simulink model "torqueBalancingPHRIStandup_WBTv5"  (Simulink 9.1)
settings: Solver=FixedStepDiscrete  StartTime=0.0  StopTime="Config.SIMULATION_TIME "  FixedStep=Config.Ts  RelTol=1e-3  EnableMultiTasking=on
StopFcn:
  | cd(fileparts(which(bdroot)));
  | stopTorqueBalancingPHRIStandup;
undefined symbols (not defined in the file or in its folder): ASSISTANT_DOF_FOR_SIMULINK, bVectorConstraintsFeet, bVectorConstraintsLegs, Config, ConstraintsMatrixFeet, ConstraintsMatrixLegs, DiscIntNeverNeededParam, Gain, Reg, ROBOT_DOF, ROBOT_DOF_FOR_SIMULINK, Sat, Sm
libraries: WBToolboxLibrary x155, simulink x5
(part 3 of 4)

== system torqueBalancingPHRIStandup_WBTv5/Robot system/Robot State and References/Internal Coordinator/Base to fixed_link ==
  qj : Inport
  inertial : Inport  Port=2
  Constant1 : Constant  Value=Config.LEFT_FOOT_IN_CONTACT_AT_0
  Constant7 : Constant  Value=eye(4)
  "LFoot to base link transform " : Subsystem
  LFoot to world transform (fixed base) : WBToolboxLibrary/Model/Kinematics/ForwardKinematics  frameName=Frames.LEFT_FOOT
      settings: SourceProductName=WholeBodyToolbox
  RFoot to world transform (fixed base) : WBToolboxLibrary/Model/Kinematics/ForwardKinematics  frameName=Frames.RIGHT_FOOT
      settings: SourceProductName=WholeBodyToolbox
  Switch : Switch  Criteria=u2 > Threshold
  fixed_LFoot_H_b : Outport
  wires:
  "LFoot to base link transform "/1(link_H_b) -> fixed_LFoot_H_b/1
  inertial/1 -> "LFoot to base link transform "/2(inertial)
  qj/1 -> "LFoot to base link transform "/1(qj), RFoot to world transform (fixed base)/2, LFoot to world transform (fixed base)/2
  Constant7/1 -> LFoot to world transform (fixed base)/1, RFoot to world transform (fixed base)/1, "LFoot to base link transform "/4(w_H_base_fixed)
  Switch/1 -> "LFoot to base link transform "/3(w_H_link)
  LFoot to world transform (fixed base)/1 -> Switch/1
  RFoot to world transform (fixed base)/1 -> Switch/3
  Constant1/1 -> Switch/2

== system torqueBalancingPHRIStandup_WBTv5/Robot system/Robot State and References/Internal Coordinator/Compute State Velocity ==
  qj : Inport
  w_H_b : Inport  Port=2
  "feetInContact " : Inport  Port=3
  Compute Base Velocity : MATLAB Function  TreatAsAtomicUnit=on
  Feet Jacobians : Subsystem
  GetMeasurement : WBToolboxLibrary/States/GetMeasurement  measuredType=Joints Velocity
      settings: SourceProductName=WholeBodyToolbox
  Mux : Mux  Inputs=2
  nu : Outport
  wires:
  GetMeasurement/1 -> Mux/2, Compute Base Velocity/4(qjDot)
  Mux/1 -> nu/1
  "feetInContact "/1 -> Compute Base Velocity/3(feetInContact)
  Compute Base Velocity/1(nu_b) -> Mux/1
  qj/1 -> Feet Jacobians/1(qj)
  w_H_b/1 -> Feet Jacobians/2(w_H_b)
  Feet Jacobians/1(J_LFoot) -> Compute Base Velocity/1(J_LeftFoot)
  Feet Jacobians/2(J_RFoot) -> Compute Base Velocity/2(J_RightFoot)

== system torqueBalancingPHRIStandup_WBTv5/Robot system/Robot State and References/Internal Coordinator/xCom ==
  w_H_b : Inport
  qj : Inport  Port=2
  CoM : WBToolboxLibrary/Model/Kinematics/ForwardKinematics  frameName=Frames.COM
      settings: SourceProductName=WholeBodyToolbox
  "CoM6D ->  CoMXYZ2" : Selector  NumberOfDimensions=2  InputPortWidth=7  IndexOptions=Index vector (dialog),Index vector (dialog)  Indices=[1 2 3],[4]  OutputSizes=1,1
  xCoM : Outport
  wires:
  qj/1 -> CoM/2
  "CoM6D ->  CoMXYZ2"/1 -> xCoM/1
  CoM/1 -> "CoM6D ->  CoMXYZ2"/1
  w_H_b/1 -> CoM/1

== system torqueBalancingPHRIStandup_WBTv5/Robot system/Robot State and References/Select State and References/Simulink Min-jerk Trajectory  ==
  CoMDes : Inport
  smoothingTimeMinJerkComDesQDes : Inport  Port=2
  MinimumJerkTrajectoryGenerator2 : WBToolboxLibrary/Utilities/MinimumJerkTrajectoryGenerator  externalSettlingTime=on  settlingTime=0.1  sampleTime=Config.Ts  resetOnSettlingTime=off  firstDerivatives=on  secondDerivatives=on  explicitInitialValue=off
      settings: SourceProductName=WholeBodyToolbox
  Mux : Mux  Inputs=3
  Selector : Selector  InputPortWidth=9  IndexOptions=Index vector (dialog)  Indices=[1 2 3]  OutputSizes=1
  Switch1 : Switch  Criteria=u2 > Threshold
  Switch3 : Switch  Criteria=u2 > Threshold
  joints.smoothingTime : Constant  Value=Sm.smoothingTimeCoM
  desired_x_dx_ddx_CoM : Outport
  wires:
  Switch1/1 -> MinimumJerkTrajectoryGenerator2/2
  MinimumJerkTrajectoryGenerator2/2 -> Mux/2
  joints.smoothingTime/1 -> Switch1/3
  Mux/1 -> Switch3/1
  Switch3/1 -> desired_x_dx_ddx_CoM/1
  smoothingTimeMinJerkComDesQDes/1 -> Switch1/1, Switch1/2, Switch3/2
  MinimumJerkTrajectoryGenerator2/3 -> Mux/3
  Selector/1 -> MinimumJerkTrajectoryGenerator2/1
  MinimumJerkTrajectoryGenerator2/1 -> Mux/1
  CoMDes/1 -> Switch3/3, Selector/1

== system torqueBalancingPHRIStandup_WBTv5/Robot system/Robot State and References/Select State and References/Visualize Gain Tuning   ==
  smoothingTimeComAndJoints : Inport
  LEFT_RIGHT_FOOT_IN_CONTACT : Inport  Port=2
  impedances : Inport  Port=3
  state : Inport  Port=4
  nu : Inport  Port=5
  Enable : EnablePort
  Demux : Demux  Outputs=2
  DoFs converter : WBToolboxLibrary/Utilities/DoFs converter  Commented=on  yarp2WBIOption=From YARP to WBI
      settings: SourceProductName=WholeBodyToolbox
  DoFs converter1 : WBToolboxLibrary/Utilities/DoFs converter  Commented=on  yarp2WBIOption=From YARP to WBI
      settings: SourceProductName=WholeBodyToolbox
  Gain : Gain  Gain=180/pi
  Gain1 : Gain  Gain=180/pi
  Impedances(t) : Scope  Commented=on  NumInputPorts=6
  Left right foot in contact : Scope
  Selector1 : Selector  InputPortWidth=6+ROBOT_DOF  IndexOptions=Index vector (dialog)  Indices=[7:6+ROBOT_DOF]  OutputSizes=1
  Selector2 : Selector  InputPortWidth=6+ROBOT_DOF  IndexOptions=Index vector (dialog)  Indices=[1:6]  OutputSizes=1
  jointsSmoothingTime : Scope  NumInputPorts=2
  linear and angular  base velocity : Scope  NumInputPorts=3
  "qjDot(t) " : Scope  Commented=on  NumInputPorts=6
  wires:
  state/1 -> "qjDot(t) "/6, linear and angular  base velocity/3, Impedances(t)/6, jointsSmoothingTime/2  "state"
  LEFT_RIGHT_FOOT_IN_CONTACT/1 -> Left right foot in contact/1  "Left right foot in contact"
  impedances/1 -> DoFs converter/1
  smoothingTimeComAndJoints/1 -> jointsSmoothingTime/1  "smoothingTimeComAndJoints"
  DoFs converter/4 -> Impedances(t)/4  "left_leg"
  DoFs converter/5 -> Impedances(t)/5  "right_leg"
  DoFs converter/3 -> Impedances(t)/3  "right_arm"
  DoFs converter/1 -> Impedances(t)/1  "torso"
  DoFs converter/2 -> Impedances(t)/2  "left_arm"
  Selector1/1 -> Gain/1
  DoFs converter1/4 -> "qjDot(t) "/4  "left_leg"
  DoFs converter1/3 -> "qjDot(t) "/3  "right_arm"
  DoFs converter1/1 -> "qjDot(t) "/1  "torso"
  DoFs converter1/2 -> "qjDot(t) "/2  "left_arm"
  nu/1 -> Selector2/1, Selector1/1
  Selector2/1 -> Demux/1
  Demux/1 -> linear and angular  base velocity/1  "vb"
  Demux/2 -> Gain1/1  "wb"
  Gain/1 -> DoFs converter1/1
  Gain1/1 -> linear and angular  base velocity/2
  DoFs converter1/5 -> "qjDot(t) "/5  "right_leg"

== system torqueBalancingPHRIStandup_WBTv5/Robot system/Robot State and References/State Machine Standup/Compute State Velocity ==
  qj : Inport
  w_H_b : Inport  Port=2
  "feetInContact " : Inport  Port=3
  "state " : Inport  Port=4
  Compute Base Velocity : MATLAB Function  TreatAsAtomicUnit=on
  Fixed Links Jacobians : Subsystem
  GetMeasurement : WBToolboxLibrary/States/GetMeasurement  measuredType=Joints Velocity
      settings: SourceProductName=WholeBodyToolbox
  Mux : Mux  Inputs=2
  nu : Outport
  wires:
  GetMeasurement/1 -> Mux/2, Compute Base Velocity/4(qjDot)
  Mux/1 -> nu/1
  "feetInContact "/1 -> Compute Base Velocity/3(feetInContact)
  Compute Base Velocity/1(nu_b) -> Mux/1
  Fixed Links Jacobians/1(J_LeftFixed) -> Compute Base Velocity/1(J_LeftFixedLink)
  Fixed Links Jacobians/2(J_RightFixed) -> Compute Base Velocity/2(J_RightFixedLink)
  "state "/1 -> Fixed Links Jacobians/1("state ")
  qj/1 -> Fixed Links Jacobians/2(qj)
  w_H_b/1 -> Fixed Links Jacobians/3(w_H_b)

== system torqueBalancingPHRIStandup_WBTv5/Robot system/Robot State and References/State Machine Standup/Compute base to fixed link transform ==
  qj : Inport
  inertial : Inport  Port=2
  Constant7 : Constant  Value=eye(4)
  "LFoot to base link transform " : Subsystem
  LFoot to world transform (fixed base) : WBToolboxLibrary/Model/Kinematics/ForwardKinematics  frameName=Frames.LEFT_FOOT
      settings: SourceProductName=WholeBodyToolbox
  LLeg to base link transform : Subsystem
  LLeg to world transform (fixed base) : WBToolboxLibrary/Model/Kinematics/ForwardKinematics  frameName=Frames.LEFT_LEG
      settings: SourceProductName=WholeBodyToolbox
  fixed_LFoot_H_b : Outport
  fixed_LLeg_H_b : Outport  Port=2
  wires:
  Constant7/1 -> LLeg to base link transform/4(w_H_base_fixed), "LFoot to base link transform "/4(w_H_base_fixed), LLeg to world transform (fixed base)/1, LFoot to world transform (fixed base)/1
  LLeg to base link transform/1(link_H_b) -> fixed_LLeg_H_b/1
  "LFoot to base link transform "/1(link_H_b) -> fixed_LFoot_H_b/1
  LFoot to world transform (fixed base)/1 -> "LFoot to base link transform "/3(w_H_link)
  LLeg to world transform (fixed base)/1 -> LLeg to base link transform/3(w_H_link)
  qj/1 -> "LFoot to base link transform "/1(qj), LLeg to base link transform/1(qj), LLeg to world transform (fixed base)/2, LFoot to world transform (fixed base)/2
  inertial/1 -> "LFoot to base link transform "/2(inertial), LLeg to base link transform/2(inertial)

== system torqueBalancingPHRIStandup_WBTv5/Robot system/Robot State and References/State Machine Standup/Visualise extrnal wrenches ==
  wL_arm : Inport
  wR_arm : Inport  Port=2
  wL_WBDT : Inport  Port=3
  wR_WBDT : Inport  Port=4
  state : Inport  Port=5
  Enable : EnablePort
  Compute current threshold : MATLAB Function  TreatAsAtomicUnit=on
  Sum : Sum  Inputs=++|
  Sum1 : Sum  Inputs=++|
  left arm ext wrench : Scope  NumInputPorts=3
  left foot ext wrench : Scope  NumInputPorts=3
  right arm ext wrench : Scope  NumInputPorts=3
  right foot ext wrench : Scope  NumInputPorts=3
  sum feet ext wrench : Scope  NumInputPorts=3
  wires:
  wR_WBDT/1 -> Sum/2, right foot ext wrench/1  "wR_WBDT"
  wL_WBDT/1 -> Sum/1, left foot ext wrench/1  "wL_WBDT"
  wR_arm/1 -> right arm ext wrench/1
  wL_arm/1 -> left arm ext wrench/1
  state/1 -> Compute current threshold/1(state), sum feet ext wrench/3, right foot ext wrench/3, left foot ext wrench/3, right arm ext wrench/3, left arm ext wrench/3
  Sum/1 -> sum feet ext wrench/1
  Sum1/1 -> sum feet ext wrench/2
  Compute current threshold/3(thresholdContactLeftFoot) -> left foot ext wrench/2, Sum1/1
  Compute current threshold/4(thresholdContactRightFoot) -> right foot ext wrench/2, Sum1/2
  Compute current threshold/1(thresholdContactLeftHand) -> left arm ext wrench/2
  Compute current threshold/2(thresholdContactRightHand) -> right arm ext wrench/2

== system torqueBalancingPHRIStandup_WBTv5/Robot system/Robot State and References/State Machine Standup/xCom ==
  w_H_b : Inport
  qj : Inport  Port=2
  CoM : WBToolboxLibrary/Model/Kinematics/ForwardKinematics  frameName=Frames.COM
      settings: SourceProductName=WholeBodyToolbox
  "CoM6D ->  CoMXYZ2" : Selector  NumberOfDimensions=2  InputPortWidth=7  IndexOptions=Index vector (dialog),Index vector (dialog)  Indices=[1 2 3],[4]  OutputSizes=1,1
  xCoM : Outport
  wires:
  qj/1 -> CoM/2
  "CoM6D ->  CoMXYZ2"/1 -> xCoM/1
  CoM/1 -> "CoM6D ->  CoMXYZ2"/1
  w_H_b/1 -> CoM/1

== system torqueBalancingPHRIStandup_WBTv5/Robot system/controller_QP/Compute angular momentum integral/Compute base to fixed link transform ==
  qj : Inport
  inertial : Inport  Port=2
  Constant7 : Constant  Value=eye(4)
  "LFoot to base link transform " : Subsystem
  LFoot to world transform (fixed base) : WBToolboxLibrary/Model/Kinematics/ForwardKinematics  frameName=Frames.LEFT_FOOT
      settings: SourceProductName=WholeBodyToolbox
  LLeg to base link transform : Subsystem
  LLeg to world transform (fixed base) : WBToolboxLibrary/Model/Kinematics/ForwardKinematics  frameName=Frames.LEFT_LEG
      settings: SourceProductName=WholeBodyToolbox
  fixed_LLeg_H_b : Outport
  fixed_LFoot_H_b : Outport  Port=2
  wires:
  Constant7/1 -> LLeg to base link transform/4(w_H_base_fixed), "LFoot to base link transform "/4(w_H_base_fixed), LLeg to world transform (fixed base)/1, LFoot to world transform (fixed base)/1
  LLeg to base link transform/1(link_H_b) -> fixed_LLeg_H_b/1
  "LFoot to base link transform "/1(link_H_b) -> fixed_LFoot_H_b/1
  LFoot to world transform (fixed base)/1 -> "LFoot to base link transform "/3(w_H_link)
  LLeg to world transform (fixed base)/1 -> LLeg to base link transform/3(w_H_link)
  qj/1 -> "LFoot to base link transform "/1(qj), LLeg to base link transform/1(qj), LLeg to world transform (fixed base)/2, LFoot to world transform (fixed base)/2
  inertial/1 -> "LFoot to base link transform "/2(inertial), LLeg to base link transform/2(inertial)

== system torqueBalancingPHRIStandup_WBTv5/Robot system/controller_QP/Compute angular momentum integral/Fixed Links Jacobians ==
  "legsInContact " : Inport
  qj : Inport  Port=2
  w_H_b : Inport  Port=3
  " " : WBToolboxLibrary/Model/Jacobians/Jacobian  frameName=Frames.LEFT_LEG
      settings: SourceProductName=WholeBodyToolbox
  "  " : WBToolboxLibrary/Model/Jacobians/Jacobian  frameName=Frames.RIGHT_LEG
      settings: SourceProductName=WholeBodyToolbox
  "   " : WBToolboxLibrary/Model/Jacobians/Jacobian  frameName=Frames.RIGHT_FOOT
      settings: SourceProductName=WholeBodyToolbox
  "       " : WBToolboxLibrary/Model/Jacobians/Jacobian  frameName=Frames.LEFT_FOOT
      settings: SourceProductName=WholeBodyToolbox
  Switch1 : Switch  Criteria=u2 > Threshold  Threshold=0.1
  Switch2 : Switch  Criteria=u2 > Threshold  Threshold=0.1
  J_LeftFixed : Outport
  J_RIghtFixed : Outport  Port=2
  wires:
  Switch2/1 -> J_RIghtFixed/1
  " "/1 -> Switch1/1
  "       "/1 -> Switch1/3
  "   "/1 -> Switch2/3
  "  "/1 -> Switch2/1
  Switch1/1 -> J_LeftFixed/1
  qj/1 -> "   "/2, "  "/2, "       "/2, " "/2
  w_H_b/1 -> "   "/1, " "/1, "       "/1, "  "/1
  "legsInContact "/1 -> Switch2/2, Switch1/2

== system torqueBalancingPHRIStandup_WBTv5/Robot system/controller_QP/Compute joint torques/QPSolver ==
  LEFT_RIGHT_FOOT_IN_CONTACT : Inport
  HessianMatrixQP1Foot : Inport  Port=2
  gradientQP1Foot : Inport  Port=3
  ConstraintsMatrixQP1Foot : Inport  Port=4
  bVectorConstraintsQP1Foot : Inport  Port=5
  HessianMatrixQP2Feet : Inport  Port=6
  gradientQP2Feet : Inport  Port=7
  ConstraintsMatrixQP2Feet : Inport  Port=8
  bVectorConstraintsQp2Feet : Inport  Port=9
  state : Inport  Port=10
  Constant1 : Constant  Value=Config.USE_QP_SOLVER
  Level-2 MATLAB S-Function : M-S-Function  FunctionName=QPBalancingStandup
  Logical Operator1 : Logic  Operator=OR  AllPortsSameDT=off  OutDataTypeStr=boolean
  ON_GAZEBO 3 : Constant  Value=Config.SCOPES_ALL
  ON_GAZEBO 4 : Constant  Value=Config.SCOPES_QP
  Visualize eventual QP failures : Subsystem
  f0OneFoot : Outport
  f0TwoFeet : Outport  Port=2
  wires:
  Level-2 MATLAB S-Function/1 -> f0TwoFeet/1
  Level-2 MATLAB S-Function/2 -> Visualize eventual QP failures/1(exitFlagQP)  "Exit flag QP two feet"
  HessianMatrixQP1Foot/1 -> Level-2 MATLAB S-Function/7
  gradientQP1Foot/1 -> Level-2 MATLAB S-Function/8
  ConstraintsMatrixQP1Foot/1 -> Level-2 MATLAB S-Function/9
  bVectorConstraintsQP1Foot/1 -> Level-2 MATLAB S-Function/10
  Level-2 MATLAB S-Function/3 -> f0OneFoot/1
  Logical Operator1/1 -> Visualize eventual QP failures/Enable
  state/1 -> Visualize eventual QP failures/2(state)
  LEFT_RIGHT_FOOT_IN_CONTACT/1 -> Level-2 MATLAB S-Function/1
  HessianMatrixQP2Feet/1 -> Level-2 MATLAB S-Function/2
  gradientQP2Feet/1 -> Level-2 MATLAB S-Function/3
  ConstraintsMatrixQP2Feet/1 -> Level-2 MATLAB S-Function/4
  bVectorConstraintsQp2Feet/1 -> Level-2 MATLAB S-Function/5
  Constant1/1 -> Level-2 MATLAB S-Function/6
  ON_GAZEBO 3/1 -> Logical Operator1/1
  ON_GAZEBO 4/1 -> Logical Operator1/2

== system torqueBalancingPHRIStandup_WBTv5/Assistant system/Real system/Dump and visualize/Assistant Data/Using Human Assistant ==
  assistant_jointData : Inport
  assistant_jointVelocitiesData : Inport  Port=2
  assistant_jointTorquesData : Inport  Port=3
  Enable : EnablePort
  Gain : Gain  Gain=180/pi
  Gain1 : Gain  Gain=180/pi
  assistant joint data : Subsystem
  assistant joint torques data : Subsystem
  assistant joint velocities data : Subsystem
  wires:
  Gain/1 -> assistant joint data/1(assistant_jointData)
  assistant_jointData/1 -> Gain/1
  Gain1/1 -> assistant joint velocities data/1(assistant_jointVelocitiesData)
  assistant_jointVelocitiesData/1 -> Gain1/1
  assistant_jointTorquesData/1 -> assistant joint torques data/1(assistant_jointTorquesData)

== system torqueBalancingPHRIStandup_WBTv5/Assistant system/Real system/Dump and visualize/Assistant Data/Using Robot Assistant ==
  assistant_jointData : Inport
  assistant_jointVelocitiesData : Inport  Port=2
  assistant_jointTorquesData : Inport  Port=3
  Enable : EnablePort
  Demux1 : Demux  Outputs=ASSISTANT_Config.numOfJointsForEachControlboard
  Demux2 : Demux  Outputs=ASSISTANT_Config.numOfJointsForEachControlboard
  Demux3 : Demux  Outputs=ASSISTANT_Config.numOfJointsForEachControlboard
  scope : Scope  NumInputPorts=5
  scope1 : Scope  NumInputPorts=5
  scope2 : Scope  NumInputPorts=5
  wires:
  Demux1/1 -> scope/1  "torso"
  Demux1/5 -> scope/5  "rightleg"
  Demux1/4 -> scope/4  "left_leg"
  assistant_jointData/1 -> Demux1/1
  Demux1/2 -> scope/2  "left_arm"
  Demux1/3 -> scope/3  "right_arm"
  Demux2/5 -> scope1/5  "rightleg"
  assistant_jointVelocitiesData/1 -> Demux2/1
  Demux2/4 -> scope1/4  "left_leg"
  Demux2/1 -> scope1/1  "torso"
  Demux2/2 -> scope1/2  "left_arm"
  Demux2/3 -> scope1/3  "right_arm"
  Demux3/5 -> scope2/5  "rightleg"
  assistant_jointTorquesData/1 -> Demux3/1
  Demux3/4 -> scope2/4  "left_leg"
  Demux3/1 -> scope2/1  "torso"
  Demux3/2 -> scope2/2  "left_arm"
  Demux3/3 -> scope2/3  "right_arm"

== system torqueBalancingPHRIStandup_WBTv5/Robot system/Robot State and References/Internal Coordinator/Base to fixed_link/LFoot to base link transform  ==
  qj : Inport
  inertial : Inport  Port=2
  w_H_link : Inport  Port=3
  w_H_base_fixed : Inport  Port=4
  Fixed base to imu transform : WBToolboxLibrary/Model/Kinematics/ForwardKinematics  frameName=Frames.IMU
      settings: SourceProductName=WholeBodyToolbox
  Fixed base to root link transform : WBToolboxLibrary/Model/Kinematics/ForwardKinematics  frameName=Frames.BASE
      settings: SourceProductName=WholeBodyToolbox
  Inv\* : Product  Inputs=/*  Multiplication=Matrix(*)
  "Inv\\*  " : Product  Inputs=/*  Multiplication=Matrix(*)
  Neck Position : WBToolboxLibrary/Utilities/YarpRead  portName=Ports.NECK_POS  signalSize=6  timeout=0.5  blocking=off  timestamp=off  autoconnect=on  errorOnConnection=off
      settings: SourceProductName=WholeBodyToolbox
  Switch6 : Switch  Criteria=u2 > Threshold
  USE_IMU4EST_BASE : Constant  Value=Config.USE_IMU4EST_BASE
  fromImuToHomogeousTransformFCN : MATLAB Function  TreatAsAtomicUnit=on
  holder 1 : WBToolboxLibrary/Utilities/holder 
      settings: SourceProductName=WholeBodyToolbox
  holder 2 : WBToolboxLibrary/Utilities/holder 
      settings: SourceProductName=WholeBodyToolbox
  neck transform : Subsystem
  link_H_b : Outport
  wires:
  Switch6/1 -> link_H_b/1
  "Inv\\*  "/1 -> Switch6/3, fromImuToHomogeousTransformFCN/3(link_H_base)  "link_H_root"
  USE_IMU4EST_BASE/1 -> Switch6/2
  Inv\*/1 -> fromImuToHomogeousTransformFCN/1(imu_H_link), holder 1/1  "imu_H_link"
  holder 2/1 -> fromImuToHomogeousTransformFCN/4(inertial_0)
  Fixed base to imu transform/1 -> Inv\*/1
  holder 1/1 -> fromImuToHomogeousTransformFCN/2(imu_H_link_0)
  qj/1 -> Fixed base to imu transform/2, Fixed base to root link transform/2
  fromImuToHomogeousTransformFCN/1(w_H_b) -> Switch6/1
  Fixed base to root link transform/1 -> "Inv\\*  "/2
  inertial/1 -> holder 2/1, fromImuToHomogeousTransformFCN/5(inertial)
  Neck Position/1 -> neck transform/1(neck port)
  neck transform/1(neck position) -> fromImuToHomogeousTransformFCN/6(neck_pos)
  w_H_link/1 -> "Inv\\*  "/1, Inv\*/2
  w_H_base_fixed/1 -> Fixed base to root link transform/1, Fixed base to imu transform/1

== system torqueBalancingPHRIStandup_WBTv5/Robot system/Robot State and References/Internal Coordinator/Compute State Velocity/Feet Jacobians ==
  qj : Inport
  w_H_b : Inport  Port=2
  Jacobian LFoot : WBToolboxLibrary/Model/Jacobians/Jacobian  frameName=Frames.LEFT_FOOT
      settings: SourceProductName=WholeBodyToolbox
  Jacobian RFoot : WBToolboxLibrary/Model/Jacobians/Jacobian  frameName=Frames.RIGHT_FOOT
      settings: SourceProductName=WholeBodyToolbox
  J_LFoot : Outport
  J_RFoot : Outport  Port=2
  wires:
  Jacobian LFoot/1 -> J_LFoot/1
  Jacobian RFoot/1 -> J_RFoot/1
  w_H_b/1 -> Jacobian RFoot/1, Jacobian LFoot/1
  qj/1 -> Jacobian LFoot/2, Jacobian RFoot/2

== system torqueBalancingPHRIStandup_WBTv5/Robot system/Robot State and References/State Machine Standup/Compute State Velocity/Fixed Links Jacobians ==
  "state " : Inport
  qj : Inport  Port=2
  w_H_b : Inport  Port=3
  " " : WBToolboxLibrary/Model/Jacobians/Jacobian  frameName=Frames.LEFT_LEG
      settings: SourceProductName=WholeBodyToolbox
  "  " : WBToolboxLibrary/Model/Jacobians/Jacobian  frameName=Frames.RIGHT_LEG
      settings: SourceProductName=WholeBodyToolbox
  "   " : WBToolboxLibrary/Model/Jacobians/Jacobian  frameName=Frames.RIGHT_FOOT
      settings: SourceProductName=WholeBodyToolbox
  "       " : WBToolboxLibrary/Model/Jacobians/Jacobian  frameName=Frames.LEFT_FOOT
      settings: SourceProductName=WholeBodyToolbox
  Constant : Constant  Value=Config.iCubStandUp
  Legs in Contact : MATLAB Function  TreatAsAtomicUnit=on
  Switch1 : Switch  Criteria=u2 > Threshold  Threshold=0.1
  Switch2 : Switch  Criteria=u2 > Threshold  Threshold=0.1
  J_LeftFixed : Outport
  J_RightFixed : Outport  Port=2
  wires:
  Switch2/1 -> J_RightFixed/1
  Legs in Contact/1(legsInContact) -> Switch2/2, Switch1/2
  " "/1 -> Switch1/1
  "       "/1 -> Switch1/3
  "   "/1 -> Switch2/3
  "  "/1 -> Switch2/1
  "state "/1 -> Legs in Contact/2(state)
  Constant/1 -> Legs in Contact/1(icubStandup)
  Switch1/1 -> J_LeftFixed/1
  qj/1 -> "   "/2, "  "/2, "       "/2, " "/2
  w_H_b/1 -> "   "/1, " "/1, "       "/1, "  "/1

== system torqueBalancingPHRIStandup_WBTv5/Robot system/Robot State and References/State Machine Standup/Compute base to fixed link transform/LFoot to base link transform  ==
  qj : Inport
  inertial : Inport  Port=2
  w_H_link : Inport  Port=3
  w_H_base_fixed : Inport  Port=4
  Fixed base to imu transform : WBToolboxLibrary/Model/Kinematics/ForwardKinematics  frameName=Frames.IMU
      settings: SourceProductName=WholeBodyToolbox
  Fixed base to root link transform : WBToolboxLibrary/Model/Kinematics/ForwardKinematics  frameName=Frames.BASE
      settings: SourceProductName=WholeBodyToolbox
  Inv\* : Product  Inputs=/*  Multiplication=Matrix(*)
  "Inv\\*  " : Product  Inputs=/*  Multiplication=Matrix(*)
  Neck Position : WBToolboxLibrary/Utilities/YarpRead  portName=Ports.NECK_POS  signalSize=6  timeout=0.5  blocking=off  timestamp=off  autoconnect=on  errorOnConnection=off
      settings: SourceProductName=WholeBodyToolbox
  Switch6 : Switch  Criteria=u2 > Threshold
  USE_IMU4EST_BASE : Constant  Value=Config.USE_IMU4EST_BASE
  fromImuToHomogeousTransformFCN : MATLAB Function  TreatAsAtomicUnit=on
  holder 1 : WBToolboxLibrary/Utilities/holder 
      settings: SourceProductName=WholeBodyToolbox
  holder 2 : WBToolboxLibrary/Utilities/holder 
      settings: SourceProductName=WholeBodyToolbox
  neck transform : Subsystem
  link_H_b : Outport
  wires:
  Switch6/1 -> link_H_b/1
  "Inv\\*  "/1 -> Switch6/3, fromImuToHomogeousTransformFCN/3(link_H_base)  "link_H_root"
  USE_IMU4EST_BASE/1 -> Switch6/2
  Inv\*/1 -> fromImuToHomogeousTransformFCN/1(imu_H_link), holder 1/1  "imu_H_link"
  holder 2/1 -> fromImuToHomogeousTransformFCN/4(inertial_0)
  Fixed base to imu transform/1 -> Inv\*/1
  holder 1/1 -> fromImuToHomogeousTransformFCN/2(imu_H_link_0)
  qj/1 -> Fixed base to imu transform/2, Fixed base to root link transform/2
  fromImuToHomogeousTransformFCN/1(w_H_b) -> Switch6/1
  Fixed base to root link transform/1 -> "Inv\\*  "/2
  inertial/1 -> holder 2/1, fromImuToHomogeousTransformFCN/5(inertial)
  Neck Position/1 -> neck transform/1(neck port)
  neck transform/1(neck position) -> fromImuToHomogeousTransformFCN/6(neck_pos)
  w_H_link/1 -> "Inv\\*  "/1, Inv\*/2
  w_H_base_fixed/1 -> Fixed base to root link transform/1, Fixed base to imu transform/1

== system torqueBalancingPHRIStandup_WBTv5/Robot system/Robot State and References/State Machine Standup/Compute base to fixed link transform/LLeg to base link transform ==
  qj : Inport
  inertial : Inport  Port=2
  w_H_link : Inport  Port=3
  w_H_base_fixed : Inport  Port=4
  Fixed base to imu transform : WBToolboxLibrary/Model/Kinematics/ForwardKinematics  frameName=Frames.IMU
      settings: SourceProductName=WholeBodyToolbox
  Fixed base to root link transform : WBToolboxLibrary/Model/Kinematics/ForwardKinematics  frameName=Frames.BASE
      settings: SourceProductName=WholeBodyToolbox
  Inv\* : Product  Inputs=/*  Multiplication=Matrix(*)
  "Inv\\*  " : Product  Inputs=/*  Multiplication=Matrix(*)
  Neck Position : WBToolboxLibrary/Utilities/YarpRead  portName=Ports.NECK_POS  signalSize=6  timeout=0.5  blocking=off  timestamp=off  autoconnect=on  errorOnConnection=off
      settings: SourceProductName=WholeBodyToolbox
  Switch6 : Switch  Criteria=u2 > Threshold
  USE_IMU4EST_BASE : Constant  Value=Config.USE_IMU4EST_BASE
  fromImuToHomogeousTransformFCN : MATLAB Function  TreatAsAtomicUnit=on
  holder 1 : WBToolboxLibrary/Utilities/holder 
      settings: SourceProductName=WholeBodyToolbox
  holder 2 : WBToolboxLibrary/Utilities/holder 
      settings: SourceProductName=WholeBodyToolbox
  neck transform : Subsystem
  link_H_b : Outport
  wires:
  Switch6/1 -> link_H_b/1
  "Inv\\*  "/1 -> Switch6/3, fromImuToHomogeousTransformFCN/3(link_H_base)  "link_H_root"
  USE_IMU4EST_BASE/1 -> Switch6/2
  Inv\*/1 -> fromImuToHomogeousTransformFCN/1(imu_H_link), holder 1/1  "imu_H_link"
  holder 2/1 -> fromImuToHomogeousTransformFCN/4(inertial_0)
  Fixed base to imu transform/1 -> Inv\*/1
  holder 1/1 -> fromImuToHomogeousTransformFCN/2(imu_H_link_0)
  qj/1 -> Fixed base to imu transform/2, Fixed base to root link transform/2
  fromImuToHomogeousTransformFCN/1(w_H_b) -> Switch6/1
  Fixed base to root link transform/1 -> "Inv\\*  "/2
  inertial/1 -> holder 2/1, fromImuToHomogeousTransformFCN/5(inertial)
  Neck Position/1 -> neck transform/1(neck port)
  neck transform/1(neck position) -> fromImuToHomogeousTransformFCN/6(neck_pos)
  w_H_link/1 -> "Inv\\*  "/1, Inv\*/2
  w_H_base_fixed/1 -> Fixed base to root link transform/1, Fixed base to imu transform/1

== system torqueBalancingPHRIStandup_WBTv5/Robot system/controller_QP/Compute angular momentum integral/Compute base to fixed link transform/LFoot to base link transform  ==
  qj : Inport
  inertial : Inport  Port=2
  w_H_link : Inport  Port=3
  w_H_base_fixed : Inport  Port=4
  Fixed base to imu transform : WBToolboxLibrary/Model/Kinematics/ForwardKinematics  frameName=Frames.IMU
      settings: SourceProductName=WholeBodyToolbox
  Fixed base to root link transform : WBToolboxLibrary/Model/Kinematics/ForwardKinematics  frameName=Frames.BASE
      settings: SourceProductName=WholeBodyToolbox
  Inv\* : Product  Inputs=/*  Multiplication=Matrix(*)
  "Inv\\*  " : Product  Inputs=/*  Multiplication=Matrix(*)
  Neck Position : WBToolboxLibrary/Utilities/YarpRead  portName=Ports.NECK_POS  signalSize=6  timeout=0.5  blocking=off  timestamp=off  autoconnect=on  errorOnConnection=off
      settings: SourceProductName=WholeBodyToolbox
  Switch6 : Switch  Criteria=u2 > Threshold
  USE_IMU4EST_BASE : Constant  Value=Config.USE_IMU4EST_BASE
  fromImuToHomogeousTransformFCN : MATLAB Function  TreatAsAtomicUnit=on
  holder 1 : WBToolboxLibrary/Utilities/holder 
      settings: SourceProductName=WholeBodyToolbox
  holder 2 : WBToolboxLibrary/Utilities/holder 
      settings: SourceProductName=WholeBodyToolbox
  neck transform : Subsystem
  link_H_b : Outport
  wires:
  Switch6/1 -> link_H_b/1
  "Inv\\*  "/1 -> Switch6/3, fromImuToHomogeousTransformFCN/3(link_H_base)  "link_H_root"
  USE_IMU4EST_BASE/1 -> Switch6/2
  Inv\*/1 -> fromImuToHomogeousTransformFCN/1(imu_H_link), holder 1/1  "imu_H_link"
  holder 2/1 -> fromImuToHomogeousTransformFCN/4(inertial_0)
  Fixed base to imu transform/1 -> Inv\*/1
  holder 1/1 -> fromImuToHomogeousTransformFCN/2(imu_H_link_0)
  qj/1 -> Fixed base to imu transform/2, Fixed base to root link transform/2
  fromImuToHomogeousTransformFCN/1(w_H_b) -> Switch6/1
  Fixed base to root link transform/1 -> "Inv\\*  "/2
  inertial/1 -> holder 2/1, fromImuToHomogeousTransformFCN/5(inertial)
  Neck Position/1 -> neck transform/1(neck port)
  neck transform/1(neck position) -> fromImuToHomogeousTransformFCN/6(neck_pos)
  w_H_link/1 -> "Inv\\*  "/1, Inv\*/2
  w_H_base_fixed/1 -> Fixed base to root link transform/1, Fixed base to imu transform/1

== system torqueBalancingPHRIStandup_WBTv5/Robot system/controller_QP/Compute angular momentum integral/Compute base to fixed link transform/LLeg to base link transform ==
  qj : Inport
  inertial : Inport  Port=2
  w_H_link : Inport  Port=3
  w_H_base_fixed : Inport  Port=4
  Fixed base to imu transform : WBToolboxLibrary/Model/Kinematics/ForwardKinematics  frameName=Frames.IMU
      settings: SourceProductName=WholeBodyToolbox
  Fixed base to root link transform : WBToolboxLibrary/Model/Kinematics/ForwardKinematics  frameName=Frames.BASE
      settings: SourceProductName=WholeBodyToolbox
  Inv\* : Product  Inputs=/*  Multiplication=Matrix(*)
  "Inv\\*  " : Product  Inputs=/*  Multiplication=Matrix(*)
  Neck Position : WBToolboxLibrary/Utilities/YarpRead  portName=Ports.NECK_POS  signalSize=6  timeout=0.5  blocking=off  timestamp=off  autoconnect=on  errorOnConnection=off
      settings: SourceProductName=WholeBodyToolbox
  Switch6 : Switch  Criteria=u2 > Threshold
  USE_IMU4EST_BASE : Constant  Value=Config.USE_IMU4EST_BASE
  fromImuToHomogeousTransformFCN : MATLAB Function  TreatAsAtomicUnit=on
  holder 1 : WBToolboxLibrary/Utilities/holder 
      settings: SourceProductName=WholeBodyToolbox
  holder 2 : WBToolboxLibrary/Utilities/holder 
      settings: SourceProductName=WholeBodyToolbox
  neck transform : Subsystem
  link_H_b : Outport
  wires:
  Switch6/1 -> link_H_b/1
  "Inv\\*  "/1 -> Switch6/3, fromImuToHomogeousTransformFCN/3(link_H_base)  "link_H_root"
  USE_IMU4EST_BASE/1 -> Switch6/2
  Inv\*/1 -> fromImuToHomogeousTransformFCN/1(imu_H_link), holder 1/1  "imu_H_link"
  holder 2/1 -> fromImuToHomogeousTransformFCN/4(inertial_0)
  Fixed base to imu transform/1 -> Inv\*/1
  holder 1/1 -> fromImuToHomogeousTransformFCN/2(imu_H_link_0)
  qj/1 -> Fixed base to imu transform/2, Fixed base to root link transform/2
  fromImuToHomogeousTransformFCN/1(w_H_b) -> Switch6/1
  Fixed base to root link transform/1 -> "Inv\\*  "/2
  inertial/1 -> holder 2/1, fromImuToHomogeousTransformFCN/5(inertial)
  Neck Position/1 -> neck transform/1(neck port)
  neck transform/1(neck position) -> fromImuToHomogeousTransformFCN/6(neck_pos)
  w_H_link/1 -> "Inv\\*  "/1, Inv\*/2
  w_H_base_fixed/1 -> Fixed base to root link transform/1, Fixed base to imu transform/1

== system torqueBalancingPHRIStandup_WBTv5/Robot system/controller_QP/Compute joint torques/QPSolver/Visualize eventual QP failures ==
  exitFlagQP : Inport
  state : Inport  Port=2
  Enable : EnablePort
  "QP status (0: no failure, 1: not using)" : Scope  NumInputPorts=2
  wires:
  exitFlagQP/1 -> "QP status (0: no failure, 1: not using)"/1  "exitFlagQP"
  state/1 -> "QP status (0: no failure, 1: not using)"/2

== system torqueBalancingPHRIStandup_WBTv5/Assistant system/Real system/Dump and visualize/Assistant Data/Using Human Assistant/assistant joint data ==
  assistant_jointData : Inport
  Scope : Scope  NumInputPorts=6
  head : Selector  InputPortWidth=66  IndexOptions=Index vector (dialog)  Indices=[16 17 18]  OutputSizes=1
  jointData : Scope  NumInputPorts=16
  left_ankle : Selector  InputPortWidth=66  IndexOptions=Index vector (dialog)  Indices=[61 62 63]  OutputSizes=1
  left_ball_foot : Selector  InputPortWidth=66  IndexOptions=Index vector (dialog)  Indices=[64 65 66]  OutputSizes=1
  left_elbow : Selector  InputPortWidth=66  IndexOptions=Index vector (dialog)  Indices=[37 38 39]  OutputSizes=1
  left_hip : Selector  InputPortWidth=66  IndexOptions=Index vector (dialog)  Indices=[55 56 57]  OutputSizes=1
  left_knee : Selector  InputPortWidth=66  IndexOptions=Index vector (dialog)  Indices=[58 59 60]  OutputSizes=1
  left_shoulder : Selector  InputPortWidth=66  IndexOptions=Index vector (dialog)  Indices=[34 35 36]  OutputSizes=1
  left_shoulder_internal : Selector  InputPortWidth=66  IndexOptions=Index vector (dialog)  Indices=[31 32 33]  OutputSizes=1
  left_wrist : Selector  InputPortWidth=66  IndexOptions=Index vector (dialog)  Indices=[40 41 42]  OutputSizes=1
  neck : Selector  InputPortWidth=66  IndexOptions=Index vector (dialog)  Indices=[13 14 15]  OutputSizes=1
  right_ankle : Selector  InputPortWidth=66  IndexOptions=Index vector (dialog)  Indices=[49 50 51]  OutputSizes=1
  right_ball_foot : Selector  InputPortWidth=66  IndexOptions=Index vector (dialog)  Indices=[52 53 54]  OutputSizes=1
  right_elbow : Selector  InputPortWidth=66  IndexOptions=Index vector (dialog)  Indices=[25 26 27]  OutputSizes=1
  right_hip : Selector  InputPortWidth=66  IndexOptions=Index vector (dialog)  Indices=[43 44 45]  OutputSizes=1
  right_knee : Selector  InputPortWidth=66  IndexOptions=Index vector (dialog)  Indices=[46 47 48]  OutputSizes=1
  right_shoulder : Selector  InputPortWidth=66  IndexOptions=Index vector (dialog)  Indices=[22 23 24]  OutputSizes=1
  right_shoulder_internal : Selector  InputPortWidth=66  IndexOptions=Index vector (dialog)  Indices=[19 20 21]  OutputSizes=1
  right_wrist : Selector  InputPortWidth=66  IndexOptions=Index vector (dialog)  Indices=[28 29 30]  OutputSizes=1
  torso_1 : Selector  InputPortWidth=66  IndexOptions=Index vector (dialog)  Indices=[10 11 12]  OutputSizes=1
  torso_2 : Selector  InputPortWidth=66  IndexOptions=Index vector (dialog)  Indices=[7 8 9]  OutputSizes=1
  torso_3 : Selector  InputPortWidth=66  IndexOptions=Index vector (dialog)  Indices=[4 5 6]  OutputSizes=1
  torso_4 : Selector  InputPortWidth=66  IndexOptions=Index vector (dialog)  Indices=[1 2 3]  OutputSizes=1
  wires:
  torso_1/1 -> jointData/1
  torso_4/1 -> jointData/4
  torso_3/1 -> jointData/3
  torso_2/1 -> jointData/2
  right_shoulder_internal/1 -> jointData/6
  left_shoulder_internal/1 -> jointData/5
  left_hip/1 -> jointData/7
  right_hip/1 -> jointData/8
  left_shoulder/1 -> jointData/9
  right_shoulder/1 -> jointData/10
  left_knee/1 -> jointData/11
  right_knee/1 -> jointData/12
  left_elbow/1 -> jointData/13
  right_elbow/1 -> jointData/14
  left_ankle/1 -> jointData/15
  right_ankle/1 -> jointData/16
  assistant_jointData/1 -> head/1, left_ball_foot/1, left_wrist/1, neck/1, right_ball_foot/1, right_wrist/1, left_shoulder/1, right_hip/1, left_hip/1, right_shoulder_internal/1, torso_1/1, torso_2/1, torso_3/1, torso_4/1, left_shoulder_internal/1, right_shoulder/1, left_knee/1, right_knee/1, left_elbow/1, right_elbow/1, right_ankle/1, left_ankle/1
  head/1 -> Scope/1
  left_ball_foot/1 -> Scope/2
  left_wrist/1 -> Scope/3
  neck/1 -> Scope/4
  right_ball_foot/1 -> Scope/5
  right_wrist/1 -> Scope/6

== system torqueBalancingPHRIStandup_WBTv5/Assistant system/Real system/Dump and visualize/Assistant Data/Using Human Assistant/assistant joint torques data ==
  assistant_jointTorquesData : Inport
  Scope : Scope  NumInputPorts=6
  head : Selector  InputPortWidth=66  IndexOptions=Index vector (dialog)  Indices=[16 17 18]  OutputSizes=1
  jointTorquesData : Scope  NumInputPorts=16
  left_ankle : Selector  InputPortWidth=66  IndexOptions=Index vector (dialog)  Indices=[61 62 63]  OutputSizes=1
  left_ball_foot : Selector  InputPortWidth=66  IndexOptions=Index vector (dialog)  Indices=[64 65 66]  OutputSizes=1
  left_elbow : Selector  InputPortWidth=66  IndexOptions=Index vector (dialog)  Indices=[37 38 39]  OutputSizes=1
  left_hip : Selector  InputPortWidth=66  IndexOptions=Index vector (dialog)  Indices=[55 56 57]  OutputSizes=1
  left_knee : Selector  InputPortWidth=66  IndexOptions=Index vector (dialog)  Indices=[58 59 60]  OutputSizes=1
  left_shoulder : Selector  InputPortWidth=66  IndexOptions=Index vector (dialog)  Indices=[34 35 36]  OutputSizes=1
  left_shoulder_internal : Selector  InputPortWidth=66  IndexOptions=Index vector (dialog)  Indices=[31 32 33]  OutputSizes=1
  left_wrist : Selector  InputPortWidth=66  IndexOptions=Index vector (dialog)  Indices=[40 41 42]  OutputSizes=1
  neck : Selector  InputPortWidth=66  IndexOptions=Index vector (dialog)  Indices=[13 14 15]  OutputSizes=1
  right_ankle : Selector  InputPortWidth=66  IndexOptions=Index vector (dialog)  Indices=[49 50 51]  OutputSizes=1
  right_ball_foot : Selector  InputPortWidth=66  IndexOptions=Index vector (dialog)  Indices=[52 53 54]  OutputSizes=1
  right_elbow : Selector  InputPortWidth=66  IndexOptions=Index vector (dialog)  Indices=[25 26 27]  OutputSizes=1
  right_hip : Selector  InputPortWidth=66  IndexOptions=Index vector (dialog)  Indices=[43 44 45]  OutputSizes=1
  right_knee : Selector  InputPortWidth=66  IndexOptions=Index vector (dialog)  Indices=[46 47 48]  OutputSizes=1
  right_shoulder : Selector  InputPortWidth=66  IndexOptions=Index vector (dialog)  Indices=[22 23 24]  OutputSizes=1
  right_shoulder_internal : Selector  InputPortWidth=66  IndexOptions=Index vector (dialog)  Indices=[19 20 21]  OutputSizes=1
  right_wrist : Selector  InputPortWidth=66  IndexOptions=Index vector (dialog)  Indices=[28 29 30]  OutputSizes=1
  torso_1 : Selector  InputPortWidth=66  IndexOptions=Index vector (dialog)  Indices=[10 11 12]  OutputSizes=1
  torso_2 : Selector  InputPortWidth=66  IndexOptions=Index vector (dialog)  Indices=[7 8 9]  OutputSizes=1
  torso_3 : Selector  InputPortWidth=66  IndexOptions=Index vector (dialog)  Indices=[4 5 6]  OutputSizes=1
  torso_4 : Selector  InputPortWidth=66  IndexOptions=Index vector (dialog)  Indices=[1 2 3]  OutputSizes=1
  wires:
  torso_1/1 -> jointTorquesData/1
  torso_4/1 -> jointTorquesData/4
  torso_3/1 -> jointTorquesData/3
  torso_2/1 -> jointTorquesData/2
  right_shoulder_internal/1 -> jointTorquesData/6
  left_shoulder_internal/1 -> jointTorquesData/5
  left_hip/1 -> jointTorquesData/7
  right_hip/1 -> jointTorquesData/8
  left_shoulder/1 -> jointTorquesData/9
  right_shoulder/1 -> jointTorquesData/10
  left_knee/1 -> jointTorquesData/11
  right_knee/1 -> jointTorquesData/12
  left_elbow/1 -> jointTorquesData/13
  right_elbow/1 -> jointTorquesData/14
  left_ankle/1 -> jointTorquesData/15
  right_ankle/1 -> jointTorquesData/16
  assistant_jointTorquesData/1 -> head/1, left_ball_foot/1, left_wrist/1, neck/1, right_ball_foot/1, right_wrist/1, left_shoulder/1, right_hip/1, left_hip/1, right_shoulder_internal/1, torso_1/1, torso_2/1, torso_3/1, torso_4/1, left_shoulder_internal/1, right_shoulder/1, left_knee/1, right_knee/1, left_elbow/1, right_elbow/1, right_ankle/1, left_ankle/1
  head/1 -> Scope/1
  left_ball_foot/1 -> Scope/2
  left_wrist/1 -> Scope/3
  neck/1 -> Scope/4
  right_ball_foot/1 -> Scope/5
  right_wrist/1 -> Scope/6

== system torqueBalancingPHRIStandup_WBTv5/Assistant system/Real system/Dump and visualize/Assistant Data/Using Human Assistant/assistant joint velocities data ==
  assistant_jointVelocitiesData : Inport
  Scope : Scope  NumInputPorts=6
  head : Selector  InputPortWidth=66  IndexOptions=Index vector (dialog)  Indices=[16 17 18]  OutputSizes=1
  jointVelocitiesData : Scope  NumInputPorts=16
  left_ankle : Selector  InputPortWidth=66  IndexOptions=Index vector (dialog)  Indices=[61 62 63]  OutputSizes=1
  left_ball_foot : Selector  InputPortWidth=66  IndexOptions=Index vector (dialog)  Indices=[64 65 66]  OutputSizes=1
  left_elbow : Selector  InputPortWidth=66  IndexOptions=Index vector (dialog)  Indices=[37 38 39]  OutputSizes=1
  left_hip : Selector  InputPortWidth=66  IndexOptions=Index vector (dialog)  Indices=[55 56 57]  OutputSizes=1
  left_knee : Selector  InputPortWidth=66  IndexOptions=Index vector (dialog)  Indices=[58 59 60]  OutputSizes=1
  left_shoulder : Selector  InputPortWidth=66  IndexOptions=Index vector (dialog)  Indices=[34 35 36]  OutputSizes=1
  left_shoulder_internal : Selector  InputPortWidth=66  IndexOptions=Index vector (dialog)  Indices=[31 32 33]  OutputSizes=1
  left_wrist : Selector  InputPortWidth=66  IndexOptions=Index vector (dialog)  Indices=[40 41 42]  OutputSizes=1
  neck : Selector  InputPortWidth=66  IndexOptions=Index vector (dialog)  Indices=[13 14 15]  OutputSizes=1
  right_ankle : Selector  InputPortWidth=66  IndexOptions=Index vector (dialog)  Indices=[49 50 51]  OutputSizes=1
  right_ball_foot : Selector  InputPortWidth=66  IndexOptions=Index vector (dialog)  Indices=[52 53 54]  OutputSizes=1
  right_elbow : Selector  InputPortWidth=66  IndexOptions=Index vector (dialog)  Indices=[25 26 27]  OutputSizes=1
  right_hip : Selector  InputPortWidth=66  IndexOptions=Index vector (dialog)  Indices=[43 44 45]  OutputSizes=1
  right_knee : Selector  InputPortWidth=66  IndexOptions=Index vector (dialog)  Indices=[46 47 48]  OutputSizes=1
  right_shoulder : Selector  InputPortWidth=66  IndexOptions=Index vector (dialog)  Indices=[22 23 24]  OutputSizes=1
  right_shoulder_internal : Selector  InputPortWidth=66  IndexOptions=Index vector (dialog)  Indices=[19 20 21]  OutputSizes=1
  right_wrist : Selector  InputPortWidth=66  IndexOptions=Index vector (dialog)  Indices=[28 29 30]  OutputSizes=1
  torso_1 : Selector  InputPortWidth=66  IndexOptions=Index vector (dialog)  Indices=[10 11 12]  OutputSizes=1
  torso_2 : Selector  InputPortWidth=66  IndexOptions=Index vector (dialog)  Indices=[7 8 9]  OutputSizes=1
  torso_3 : Selector  InputPortWidth=66  IndexOptions=Index vector (dialog)  Indices=[4 5 6]  OutputSizes=1
  torso_4 : Selector  InputPortWidth=66  IndexOptions=Index vector (dialog)  Indices=[1 2 3]  OutputSizes=1
  wires:
  torso_1/1 -> jointVelocitiesData/1
  torso_4/1 -> jointVelocitiesData/4
  torso_3/1 -> jointVelocitiesData/3
  torso_2/1 -> jointVelocitiesData/2
  right_shoulder_internal/1 -> jointVelocitiesData/6
  left_shoulder_internal/1 -> jointVelocitiesData/5
  left_hip/1 -> jointVelocitiesData/7
  right_hip/1 -> jointVelocitiesData/8
  left_shoulder/1 -> jointVelocitiesData/9
  right_shoulder/1 -> jointVelocitiesData/10
  left_knee/1 -> jointVelocitiesData/11
  right_knee/1 -> jointVelocitiesData/12
  left_elbow/1 -> jointVelocitiesData/13
  right_elbow/1 -> jointVelocitiesData/14
  left_ankle/1 -> jointVelocitiesData/15
  right_ankle/1 -> jointVelocitiesData/16
  assistant_jointVelocitiesData/1 -> head/1, left_ball_foot/1, left_wrist/1, neck/1, right_ball_foot/1, right_wrist/1, left_shoulder/1, right_hip/1, left_hip/1, right_shoulder_internal/1, torso_1/1, torso_2/1, torso_3/1, torso_4/1, left_shoulder_internal/1, right_shoulder/1, left_knee/1, right_knee/1, left_elbow/1, right_elbow/1, right_ankle/1, left_ankle/1
  head/1 -> Scope/1
  left_ball_foot/1 -> Scope/2
  left_wrist/1 -> Scope/3
  neck/1 -> Scope/4
  right_ball_foot/1 -> Scope/5
  right_wrist/1 -> Scope/6

== system torqueBalancingPHRIStandup_WBTv5/Robot system/Robot State and References/Internal Coordinator/Base to fixed_link/LFoot to base link transform /neck transform ==
  neck port : Inport
  Constant : Constant  Value=zeros(3,1)
  Gain : Gain  Gain=pi/180
  Selector1 : Selector  InputPortWidth=6  IndexOptions=Index vector (dialog)  Indices=[1:3]  OutputSizes=1
  Switch : Switch  Criteria=u2 > Threshold
  USE_IMU4EST_BASE1 : Constant  Value=Config.CORRECT_NECK_IMU
  neck position : Outport
  wires:
  neck port/1 -> Gain/1
  USE_IMU4EST_BASE1/1 -> Switch/2
  Switch/1 -> neck position/1
  Gain/1 -> Selector1/1
  Constant/1 -> Switch/3
  Selector1/1 -> Switch/1  "neck pos"

== system torqueBalancingPHRIStandup_WBTv5/Robot system/Robot State and References/State Machine Standup/Compute base to fixed link transform/LFoot to base link transform /neck transform ==
  neck port : Inport
  Constant : Constant  Value=zeros(3,1)
  Gain : Gain  Gain=pi/180
  Selector1 : Selector  InputPortWidth=6  IndexOptions=Index vector (dialog)  Indices=[1:3]  OutputSizes=1
  Switch : Switch  Criteria=u2 > Threshold
  USE_IMU4EST_BASE1 : Constant  Value=Config.CORRECT_NECK_IMU
  neck position : Outport
  wires:
  neck port/1 -> Gain/1
  USE_IMU4EST_BASE1/1 -> Switch/2
  Switch/1 -> neck position/1
  Gain/1 -> Selector1/1
  Constant/1 -> Switch/3
  Selector1/1 -> Switch/1  "neck pos"

== system torqueBalancingPHRIStandup_WBTv5/Robot system/Robot State and References/State Machine Standup/Compute base to fixed link transform/LLeg to base link transform/neck transform ==
  neck port : Inport
  Constant : Constant  Value=zeros(3,1)
  Gain : Gain  Gain=pi/180
  Selector1 : Selector  InputPortWidth=6  IndexOptions=Index vector (dialog)  Indices=[1:3]  OutputSizes=1
  Switch : Switch  Criteria=u2 > Threshold
  USE_IMU4EST_BASE1 : Constant  Value=Config.CORRECT_NECK_IMU
  neck position : Outport
  wires:
  neck port/1 -> Gain/1
  USE_IMU4EST_BASE1/1 -> Switch/2
  Switch/1 -> neck position/1
  Gain/1 -> Selector1/1
  Constant/1 -> Switch/3
  Selector1/1 -> Switch/1  "neck pos"

== system torqueBalancingPHRIStandup_WBTv5/Robot system/controller_QP/Compute angular momentum integral/Compute base to fixed link transform/LFoot to base link transform /neck transform ==
  neck port : Inport
  Constant : Constant  Value=zeros(3,1)
  Gain : Gain  Gain=pi/180
  Selector1 : Selector  InputPortWidth=6  IndexOptions=Index vector (dialog)  Indices=[1:3]  OutputSizes=1
  Switch : Switch  Criteria=u2 > Threshold
  USE_IMU4EST_BASE1 : Constant  Value=Config.CORRECT_NECK_IMU
  neck position : Outport
  wires:
  neck port/1 -> Gain/1
  USE_IMU4EST_BASE1/1 -> Switch/2
  Switch/1 -> neck position/1
  Gain/1 -> Selector1/1
  Constant/1 -> Switch/3
  Selector1/1 -> Switch/1  "neck pos"

== system torqueBalancingPHRIStandup_WBTv5/Robot system/controller_QP/Compute angular momentum integral/Compute base to fixed link transform/LLeg to base link transform/neck transform ==
  neck port : Inport
  Constant : Constant  Value=zeros(3,1)
  Gain : Gain  Gain=pi/180
  Selector1 : Selector  InputPortWidth=6  IndexOptions=Index vector (dialog)  Indices=[1:3]  OutputSizes=1
  Switch : Switch  Criteria=u2 > Threshold
  USE_IMU4EST_BASE1 : Constant  Value=Config.CORRECT_NECK_IMU
  neck position : Outport
  wires:
  neck port/1 -> Gain/1
  USE_IMU4EST_BASE1/1 -> Switch/2
  Switch/1 -> neck position/1
  Gain/1 -> Selector1/1
  Constant/1 -> Switch/3
  Selector1/1 -> Switch/1  "neck pos"

== matlab function Robot system/controller_QP/Compute angular momentum integral/Compute base to fixed link transform/LFoot to base link transform /fromImuToHomogeousTransformFCN ==
  data: imu_H_link input double; imu_H_link_0 input double; link_H_base input double; inertial_0 input double; inertial input double; neck_pos input double; w_H_b output double; Config parameter double
function w_H_b = worldToBaseTransformWithIMUFCN(imu_H_link,imu_H_link_0,link_H_base,inertial_0,inertial,neck_pos,Config)

    w_H_b = worldToBaseTransformWithIMU(imu_H_link,imu_H_link_0,link_H_base,inertial_0,inertial,neck_pos,Config);

end

== matlab function Robot system/Robot State and References/Internal Coordinator/Base to fixed_link/LFoot to base link transform /fromImuToHomogeousTransformFCN ==
  data: imu_H_link input double; imu_H_link_0 input double; link_H_base input double; inertial_0 input double; inertial input double; neck_pos input double; w_H_b output double; Config parameter double
function w_H_b = worldToBaseTransformWithIMUFCN(imu_H_link,imu_H_link_0,link_H_base,inertial_0,inertial,neck_pos,Config)

    w_H_b = worldToBaseTransformWithIMU(imu_H_link,imu_H_link_0,link_H_base,inertial_0,inertial,neck_pos,Config);

end

== matlab function Robot system/Robot State and References/State Machine Standup/Compute base to fixed link transform/LLeg to base link transform/fromImuToHomogeousTransformFCN ==
  data: imu_H_link input double; imu_H_link_0 input double; link_H_base input double; inertial_0 input double; inertial input double; neck_pos input double; w_H_b output double; Config parameter double
function w_H_b = worldToBaseTransformWithIMUFCN(imu_H_link,imu_H_link_0,link_H_base,inertial_0,inertial,neck_pos,Config)

    w_H_b = worldToBaseTransformWithIMU(imu_H_link,imu_H_link_0,link_H_base,inertial_0,inertial,neck_pos,Config);

end

== matlab function Robot system/controller_QP/Compute angular momentum integral/Compute base to fixed link transform/LLeg to base link transform/fromImuToHomogeousTransformFCN ==
  data: imu_H_link input double; imu_H_link_0 input double; link_H_base input double; inertial_0 input double; inertial input double; neck_pos input double; w_H_b output double; Config parameter double
function w_H_b = worldToBaseTransformWithIMUFCN(imu_H_link,imu_H_link_0,link_H_base,inertial_0,inertial,neck_pos,Config)

    w_H_b = worldToBaseTransformWithIMU(imu_H_link,imu_H_link_0,link_H_base,inertial_0,inertial,neck_pos,Config);

end
